simulink model "NeuronalModelDetector"  (R2016b)
settings: Solver=FixedStepDiscrete  StartTime=0.0  StopTime=inf  FixedStep=sCoreParams.core.stepPeriod  RelTol=1e-3  EnableMultiTasking=on
undefined symbols (not defined in the file): High, Low, neuralModelParams, sCoreParams
libraries: dspswit3 x5, simulink x2
settings Model: Creator=anish  LastModifiedBy=rzelmann
settings SolverCC: EnableConcurrentExecution=on  ConcurrentTasks=on
settings DataIOCC: SaveFormat=StructureWithTime  SignalLoggingSaveFormat=ModelDataLogs  SaveOutput=off  SignalLogging=off  DSMLogging=off  SaveTime=off
settings OptimizationCC: BlockReduction=off  ConditionallyExecuteInputs=off  DefaultParameterBehavior=Inlined  OptimizeBlockIOStorage=off  BufferReuse=off  GlobalBufferReuse=off  ExpressionFolding=off  LocalBlockOutputs=off  LifeSpan=inf
settings DebuggingCC: SignalRangeChecking=error  SaveWithParameterizedLinksMsg=none  AllowSymbolicDim=off  ModelReferenceSymbolNameMessage=none  StateNameClashWarn=warning  SFUnexpectedBacktrackingDiag=warning  SFNoUnconditionalDefaultTransitionDiag=warning  SFExecutionAtInitializationDiag=none
settings HardwareCC: ProdBitPerPointer=32  ProdBitPerSizeT=32  ProdBitPerPtrDiffT=32  ProdLargestAtomicFloat=None  ProdWordSize=32  ProdLongLongMode=on  ProdHWDeviceType=Generic->32-bit x86 compatible  TargetBitPerPointer=64  TargetLargestAtomicFloat=Float  TargetLongLongMode=on  TargetIntDivRoundTo=Zero  TargetEndianess=LittleEndian  TargetWordSize=64  TargetHWDeviceType=Intel->x86-64 (Windows64)
settings ModelReferenceCC: UpdateModelReferenceTargets=Force  ModelReferenceNumInstancesAllowed=Single  ModelReferencePassRootInputsByReference=off
settings RTWCC: SystemTargetFile=slrt.tlc  TemplateMakefile=slrt_default_tmf  Description=Simulink Real-Time  BuildConfiguration=Faster Runs  RTWCompilerOptimization=on
settings ConfigComp: CovMetricSettings=dw  CovHtmlReporting=on  CovSaveCumulativeToWorkspaceVar=on  CovSaveSingleToWorkspaceVar=on  CovExternalEMLEnable=off  CovSFcnEnable=off

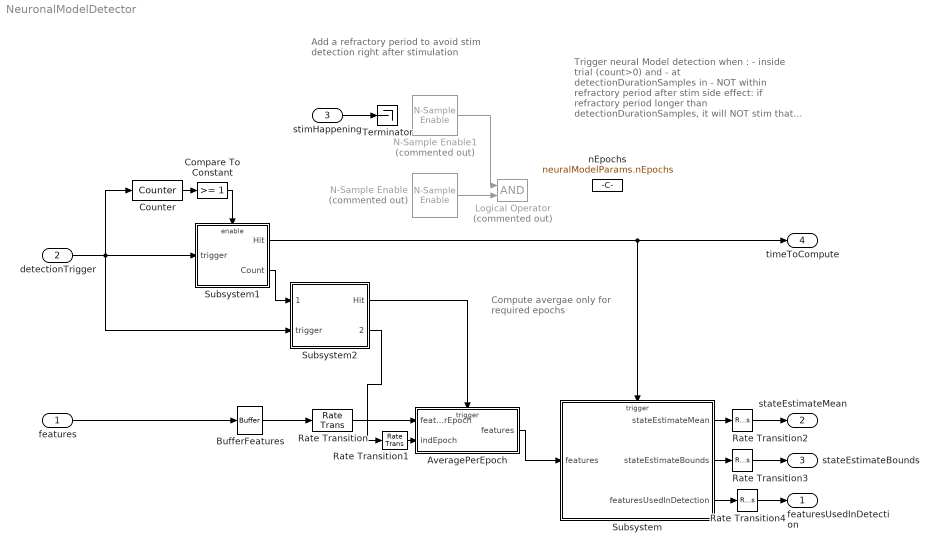
== system NeuronalModelDetector ==
  note: Compute avergae only
      |  for required epochs
  note: Trigger neural Model detection when :
      |  -  inside trial (count>0) and
      | -  at detectionDurationSamples in
      | - NOT within refractory period after stim
      | side effect: if refractory period longer than detectionDurationSamples, it will NOT stim that next trial
  note: Add a refractory period to avoid
      | stim detection right after stimulation
  features : Inport  PortDimensions=[1 neuralModelParams.nFeaturesPerEpoch]
  detectionTrigger : Inport  Port=2  OutDataTypeStr=boolean  SampleTime=sCoreParams.core.stepPeriod
  stimHappening : Inport  Port=3  OutDataTypeStr=boolean  SampleTime=sCoreParams.core.stepPeriod
  AveragePerEpoch : Subsystem
  BufferFeatures : Buffer  N=floor(sCoreParams.decoders.txDetector.detectionDurationSteps / neuralModelParams.nEpochs)  V=floor(sCoreParams.decoders.txDetector.detectionDurationSteps / neuralModelParams.nEpochs) - 1  TreatMby1Signals=One channel  OutputFrames=off
  Compare To Constant : simulink/Logic and Bit Operations/Compare To Constant  relop=>=  const=1  OutDataTypeStr=boolean
  Counter : dspswit3/Counter  Direction=Up  CountEvent=Rising edge  CounterSize=32 bits  MaxCount=sCoreParams.decoders.txDetector.detectionDurationSamples *5  InitialCount=0  Output=Count  HitValue=sCoreParams.decoders.txDetector.detectionDurationSamples  ResetInput=off  SamplesPerFrame=1  Ts=-1  CntDtype=double  HitDtype=Logical
  Logical Operator : Logic  Commented=on  IconShape=distinctive  AllPortsSameDT=off  OutDataTypeStr=boolean
  N-Sample Enable : dspswit3/N-Sample Enable  Commented=on  N=sCoreParams.decoders.txDetector.detectionDurationSamples  ActiveLevel=Low (0)  reset=on  TriggerType=Non-zero sample  Ts=1  DataType=Logical
  N-Sample Enable1 : dspswit3/N-Sample Enable  Commented=on  N=sCoreParams.decoders.txDetector.delayAfterStimSamples  ActiveLevel=High (1)  reset=on  TriggerType=Rising edge  Ts=1  DataType=Logical
  Rate Transition{,1..4} (5 alike) : RateTransition
  Subsystem : Subsystem
  Subsystem1 : Subsystem
  Subsystem2 : Subsystem
  Terminator : Terminator
  nEpochs : Constant  Value=neuralModelParams.nEpochs
  featuresUsedInDetection : Outport  PortDimensions=[1 neuralModelParams.nFeatures]
  stateEstimateMean : Outport  Port=2  PortDimensions=1
  stateEstimateBounds : Outport  Port=3  PortDimensions=[1 2]
  timeToCompute : Outport  Port=4  PortDimensions=1
  wires:
  features/1 -> BufferFeatures/1
  Subsystem/1(stateEstimateMean) -> Rate Transition2/1
  BufferFeatures/1 -> Rate Transition/1
  N-Sample Enable1/1 -> Logical Operator/1
  stimHappening/1 -> Terminator/1
  detectionTrigger/1 -> Subsystem2/2(trigger), Subsystem1/1(trigger), Counter/1
  N-Sample Enable/1 -> Logical Operator/2
  Subsystem/3(featuresUsedInDetection) -> Rate Transition4/1
  Subsystem/2(stateEstimateBounds) -> Rate Transition3/1
  Subsystem1/1(Hit) -> timeToCompute/1, Subsystem/Trigger
  Subsystem1/2(Count) -> Subsystem2/1(timeInTrial)
  Subsystem2/1(Hit) -> AveragePerEpoch/Trigger
  Compare To Constant/1 -> Subsystem1/Enable
  Counter/1 -> Compare To Constant/1
  Rate Transition/1 -> AveragePerEpoch/1(featuresPerEpoch)
  Rate Transition1/1 -> AveragePerEpoch/2(indEpoch)
  Subsystem2/2(indEpoch) -> Rate Transition1/1
  AveragePerEpoch/1(features) -> Subsystem/1(features)
  Rate Transition2/1 -> stateEstimateMean/1
  Rate Transition3/1 -> stateEstimateBounds/1
  Rate Transition4/1 -> featuresUsedInDetection/1

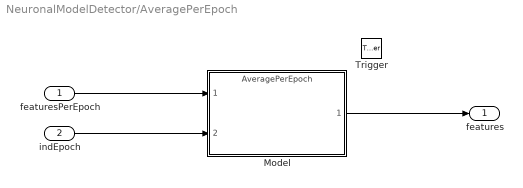
== system NeuronalModelDetector/AveragePerEpoch ==
  featuresPerEpoch : Inport
  indEpoch : Inport  Port=2
  Trigger : TriggerPort  VariantControl=Variant  PortDimensions=1
  Model : ModelReference  ModelNameDialog=AveragePerEpoch.slx  SimulationMode=Normal  ModelReferenceVersion=1.490
  features : Outport  PortDimensions=[1 neuralModelParams.nFeatures]
  wires:
  indEpoch/1 -> Model/2
  Model/1 -> features/1
  featuresPerEpoch/1 -> Model/1

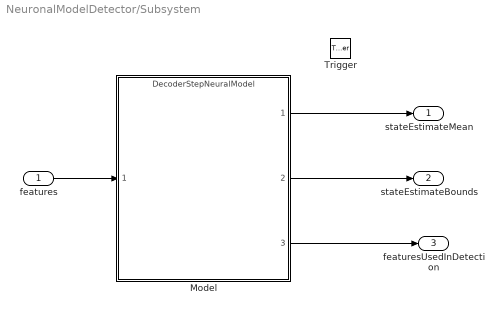
== system NeuronalModelDetector/Subsystem ==
  features : Inport  PortDimensions=[1 neuralModelParams.nFeatures]
  Trigger : TriggerPort  VariantControl=Variant  PortDimensions=1
  Model : ModelReference  ModelNameDialog=DecoderStepNeuralModel.slx  SimulationMode=Normal  ModelReferenceVersion=1.492
  stateEstimateMean : Outport  InitialOutput=-500
  stateEstimateBounds : Outport  Port=2  InitialOutput=[-500 -500]
  featuresUsedInDetection : Outport  Port=3
  wires:
  features/1 -> Model/1
  Model/3 -> featuresUsedInDetection/1
  Model/2 -> stateEstimateBounds/1
  Model/1 -> stateEstimateMean/1

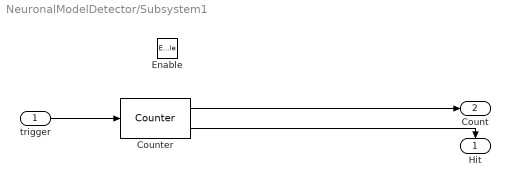
== system NeuronalModelDetector/Subsystem1 ==
  trigger : Inport
  Enable : EnablePort
  Counter : dspswit3/Counter  Direction=Up  CountEvent=Free running  CounterSize=32 bits  MaxCount=sCoreParams.decoders.txDetector.detectionDurationSamples *5  InitialCount=1  Output=Count and Hit  HitValue=sCoreParams.decoders.txDetector.detectionDurationSteps  ResetInput=on  SamplesPerFrame=1  Ts=-1  CntDtype=double  HitDtype=Logical
  Hit : Outport
  Count : Outport  Port=2  InitialOutput=1
  wires:
  Counter/1 -> Count/1
  Counter/2 -> Hit/1
  trigger/1 -> Counter/1

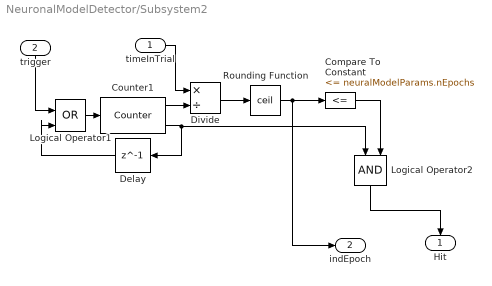
== system NeuronalModelDetector/Subsystem2 ==
  timeInTrial : Inport
  trigger : Inport  Port=2
  Compare To Constant : simulink/Logic and Bit Operations/Compare To Constant  relop=<=  const=neuralModelParams.nEpochs  OutDataTypeStr=boolean
  Counter1 : dspswit3/Counter  Direction=Up  CountEvent=Free running  CounterSize=32 bits  MaxCount=sCoreParams.decoders.txDetector.detectionDurationSamples *5  InitialCount=1  Output=Count and Hit  HitValue=floor(sCoreParams.decoders.txDetector.detectionDurationSteps/neuralModelParams.nEpochs)  ResetInput=on  SamplesPerFrame=1  Ts=-1  CntDtype=double  HitDtype=Logical
  Delay : Delay  DelayLength=1
  Divide : Product  Inputs=*/
  Logical Operator1 : Logic  Operator=OR  IconShape=distinctive  AllPortsSameDT=off  OutDataTypeStr=boolean
  Logical Operator2 : Logic  IconShape=distinctive  AllPortsSameDT=off  OutDataTypeStr=boolean
  Rounding Function : Rounding  Operator=ceil
  Hit : Outport
  indEpoch : Outport  Port=2
  wires:
  Logical Operator2/1 -> Hit/1
  Divide/1 -> Rounding Function/1
  Rounding Function/1 -> indEpoch/1, Compare To Constant/1
  Logical Operator1/1 -> Counter1/1
  Delay/1 -> Logical Operator1/2
  Compare To Constant/1 -> Logical Operator2/2
  Counter1/2 -> Logical Operator2/1, Delay/1
  Counter1/1 -> Divide/2
  timeInTrial/1 -> Divide/1
  trigger/1 -> Logical Operator1/1
